simulink model "stateflow_playground"  (R2024a)
settings: Solver=VariableStepAuto  StartTime=0.0  StopTime=0.001  RelTol=1e-3
values from neighbouring files (symbols this model uses):
  Ts = 1/Fs    (= 7.50007500075e-06)    [new_generation_coeff.m]    (also in simon_test.m; simple_fft_test.m = 1/F; testPSD_c2d.m; testPSD_simulink.m)
libraries: simulink_extras x1
settings Model: Creator=Simon  LastModifiedBy=Simon

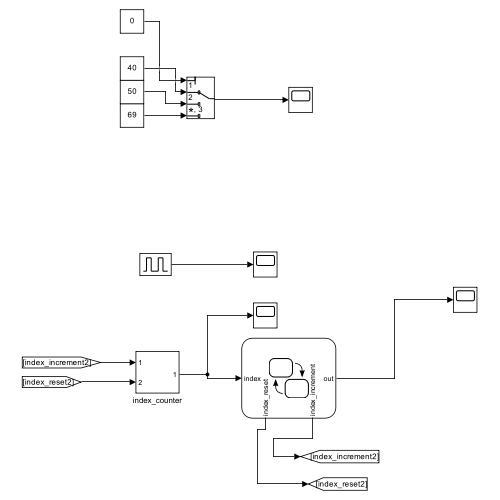
[thumbnail: Simulink's stored preview of the top-level diagram]
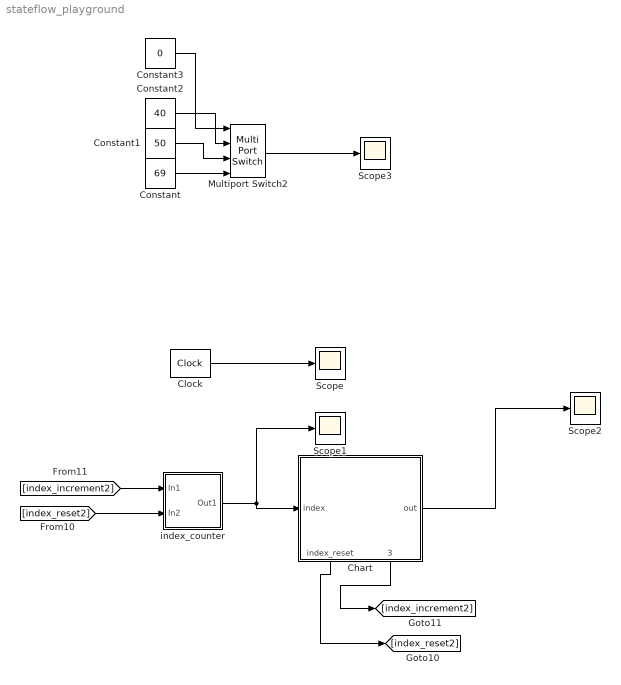
== system stateflow_playground ==
  Chart : Stateflow chart  TreatAsAtomicUnit=on
      settings: PortSchema="{\"entries\":[{\"content\":{\"sides\":[{\"content\":{\"connectorIds\":[\"In1\"]},\"type\":\"ConnectorPlacement.EquallySpacedRectSide\",\"uuid\":\"9bc4e325-a2e2-4b80-9835-b05134aae33d\"},{\"content\":{\"connectorIds\":[\"Out1\"],\"side\":\"RIGHT\"},\"type\":\"ConnectorPlacement.EquallySpacedRectSide\",\"uuid\":\"51d4be82-dc76-4d5f-a5e6-dc6c647b6448\"},{\"content\":{\"side\":\"TOP\"},\"type\":\"ConnectorPlacement.EquallySpacedRectSide\",\"uuid\":\"e49ab8ad-e9e9-45fb-91df-07b66341b83a\"},{\"content\":{\"connectorIds\":[\"Out2\",\"Out3\"],\"side\":\"BOTTOM\"},\"type\":\"ConnectorPlacement.EquallySpacedRectSide\",\"uuid\":\"8c52c93f-8960-4481-8f5d-610f415e25f4\"}]},\"type\":\"ConnectorPlacement.EquallySpacedConnector\",\"uuid\":\"1d12acf1-081a-49f0-8fa2-75453588923b\"}],\"packageUris\":[\"http://schema.mathworks.com/mf0/Connector/R2020b\"],\"version\":\"1.0\"}"
  Clock : simulink_extras/Flip Flops/Clock  period=Ts
  Constant : Constant  Value=69
  Constant1 : Constant  Value=50
  Constant2 : Constant  Value=40
  Constant3 : Constant  Value=0
  Multiport Switch2 : MultiPortSwitch  DiagnosticForDefault=None  SaturateOnIntegerOverflow=off  InputSameDT=off
  Scope{,1..3} (4 alike) : Scope
  index_counter : Subsystem
  wires:
  index_counter/1(Out1) -> Scope1/1, Chart/1(index)
  [index_increment2] -> index_counter/1(In1)
  [index_reset2] -> index_counter/2(In2)
  Chart/3(index_increment) -> [index_increment2]
  Chart/2(index_reset) -> [index_reset2]
  Clock/1 -> Scope/1
  Chart/1(out) -> Scope2/1
  Constant/1 -> Multiport Switch2/4
  Constant1/1 -> Multiport Switch2/3
  Constant2/1 -> Multiport Switch2/2
  Constant3/1 -> Multiport Switch2/1
  Multiport Switch2/1 -> Scope3/1

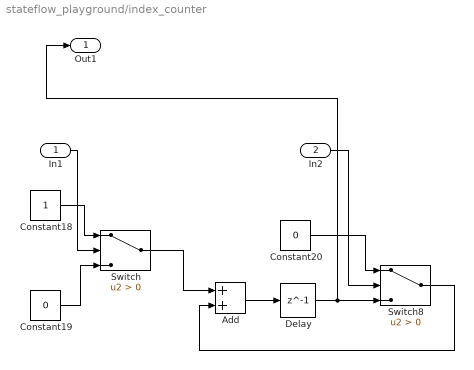
== system stateflow_playground/index_counter ==
  In1 : Inport
  In2 : Inport  Port=2
  Add : Sum  OutDataTypeStr=fixdt(0,4,0)  AccumDataTypeStr=fixdt(0,4,0)
  Constant18 : Constant  OutDataTypeStr=fixdt(0,8,0)  SampleTime=Ts
  Constant19 : Constant  Value=0  OutDataTypeStr=fixdt(0,8,0)  SampleTime=Ts
  Constant20 : Constant  Value=0  OutDataTypeStr=fixdt(0,8,0)  SampleTime=Ts
  Delay : Delay  DelayLength=1  InitialCondition=0  SampleTime=Ts
  Switch : Switch  Criteria=u2 > Threshold  OutDataTypeStr=fixdt(0,8,0)  SaturateOnIntegerOverflow=off  InputSameDT=off
  Switch8 : Switch  Criteria=u2 > Threshold  OutDataTypeStr=fixdt(0,8,0)  SaturateOnIntegerOverflow=off  InputSameDT=off
  Out1 : Outport
  wires:
  Constant19/1 -> Switch/3
  Switch8/1 -> Add/2
  Switch/1 -> Add/1
  Delay/1 -> Out1/1, Switch8/3
  In2/1 -> Switch8/2
  Add/1 -> Delay/1
  Constant20/1 -> Switch8/1
  Constant18/1 -> Switch/1
  In1/1 -> Switch/2

== stateflow chart stateflow_playground/Chart ==
  state initial_state
    during:
    index_reset = 1;
    index_increment = 0;
    %exit:
    %index_increment = 1;
  state lol
    %entry:
    %index_increment = 1;
  state enable_state
    entry:
    index_increment = 1;
    out = index;
    exit:
    out = 0;
  state test
    entry:
    index_reset = 1;
    out = index
    exit:
    index_reset = 0;
    out = 0;
  (default) -> initial_state
  initial_state -> lol
  lol -> enable_state
  test -> enable_state
  enable_state -> test : [index == 4]
  data: out output; index input; index_reset output; index_increment output
